simulink model "ADCS_loop"  (R2026a)
settings: Solver=FixedStepDiscrete  StopTime=1500  FixedStep=0.05  EnableMultiTasking=on
undefined symbols (not defined in the file): abs_omega, abs_q, area_of_coil, DiscIntNeverNeededParam, ECI_orbit_positions, k_gain_mag, MOI_tensor, mu_eff, no_of_turns, q_demanded, wheel_omega_initial
libraries: matrix_library x4, dspinverses x1, vrlib x1, dspbuff3 x1
settings Model: Creator=CS  LastModifiedBy=CS
settings SolverCC: AllowMultiTaskInputOutput=on

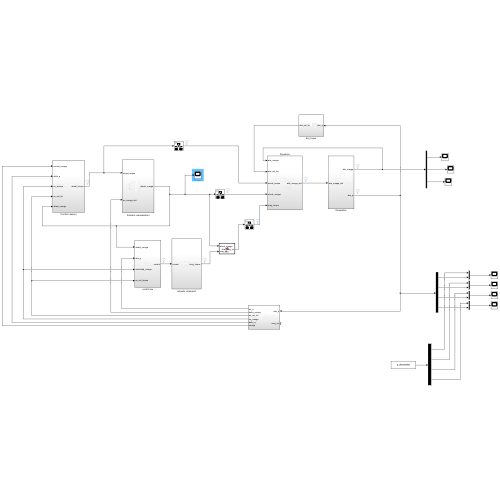
[thumbnail: Simulink's stored preview of the top-level diagram]
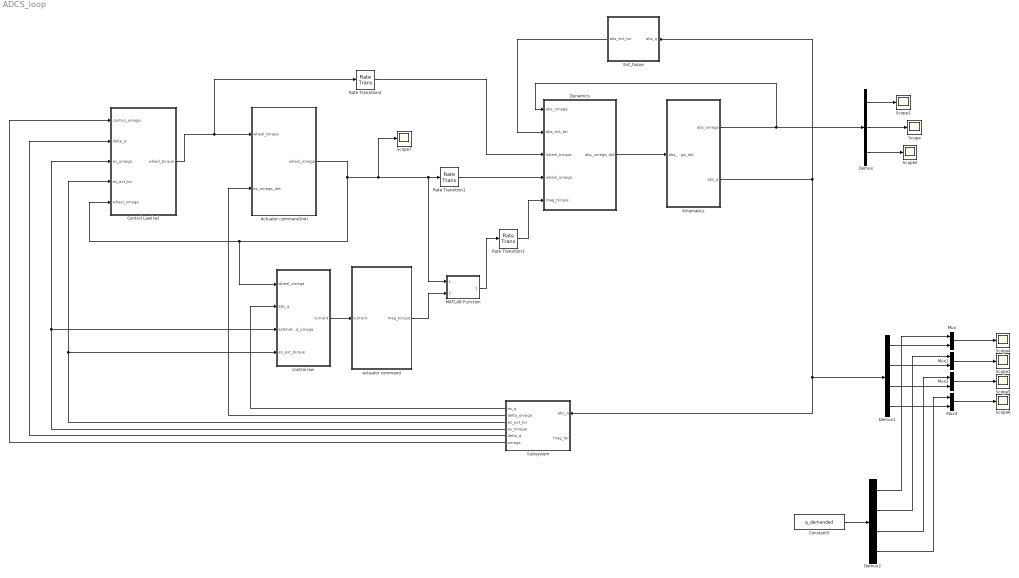
== system ADCS_loop ==
  Actuator command(rw) : Subsystem
  Constant5 : Constant  Value=q_demanded
  Control Law(rw) : Subsystem
  Demux : Demux  Outputs=3
  Demux1 : Demux
  Demux2 : Demux
  Dynamics : Subsystem
  Ext_toque : Subsystem
  Kinematics : Subsystem
  MATLAB Function : MATLAB Function  TreatAsAtomicUnit=on  SystemSampleTime=0.2
  Mux{,1..3} (4 alike) : Mux  Inputs=2
  Rate Transition1 : RateTransition  OutPortSampleTime=0.05
  Rate Transition2 : RateTransition  OutPortSampleTime=0.05
  Rate Transition3 : RateTransition  OutPortSampleTime=0.05
  Scope{,1..7} (8 alike) : Scope
      Scope settings: ActiveDisplayYMinimum=-0.10145714218919644  ActiveDisplayYMaximum=0.1169019272618283
      Scope1 settings: ActiveDisplayYMinimum=-0.0061261723528138138  ActiveDisplayYMaximum=0.0036565085131540572
      Scope2 settings: ActiveDisplayYMinimum=-0.24985187557912408  ActiveDisplayYMaximum=0.81416779259021288  DataLoggingVariableName=ScopeData2
      Scope3 settings: ActiveDisplayYMinimum=-0.0068417213457600129  ActiveDisplayYMaximum=0.0019405957953945842  DataLoggingVariableName=ScopeData3
      Scope4 settings: ActiveDisplayYMinimum=-0.11784086534209379  ActiveDisplayYMaximum=0.16507427528637539  DataLoggingVariableName=ScopeData4
      Scope5 settings: ActiveDisplayYMinimum=0.6667269446379438  ActiveDisplayYMaximum=0.9454278732496123  DataLoggingVariableName=ScopeData5
      Scope6 settings: ActiveDisplayYMinimum=0.44158444098494709  ActiveDisplayYMaximum=0.4580946893794699  DataLoggingVariableName=ScopeData6
      Scope7 settings: ActiveDisplayYMinimum=-2840.1232496648549  ActiveDisplayYMaximum=7000.2332954035792  DataLoggingVariableName=ScopeData7
  Subsystem : Subsystem
  actuator command : Subsystem
  control law : Subsystem
  wires:
  Rate Transition1/1 -> Dynamics/4(wheel_omega)
  Kinematics/2(abs_q) -> Subsystem/1(abs_q), Demux1/1, Ext_toque/1(abs_q)
  Dynamics/1(abs_omega_dot) -> Kinematics/1(abs_omega_dot)
  Kinematics/1(abs_omega) -> Demux/1, Dynamics/1(abs_omega)
  Demux/2 -> Scope/1
  Demux/3 -> Scope2/1
  Demux/1 -> Scope3/1
  Control Law(rw)/1(wheel_torque) -> Rate Transition2/1, Actuator command(rw)/1(wheel_torque)
  Actuator command(rw)/1(wheel_omega) -> control law/1(wheel_omega), Control Law(rw)/5(wheel_omega), Scope7/1, Rate Transition1/1, MATLAB Function/1(wheel_omega)
  Rate Transition2/1 -> Dynamics/3(wheel_torque)
  Constant5/1 -> Demux2/1
  Demux1/1 -> Mux/2
  Demux2/1 -> Mux/1
  Demux1/2 -> Mux1/2
  Demux2/2 -> Mux1/1
  Demux1/3 -> Mux2/2
  Demux2/3 -> Mux2/1
  Mux3/1 -> Scope6/1
  Demux1/4 -> Mux3/2
  Demux2/4 -> Mux3/1
  Mux2/1 -> Scope5/1
  Mux1/1 -> Scope1/1
  Mux/1 -> Scope4/1
  Ext_toque/1(abs_ext_tor) -> Dynamics/2(abs_ext_tor)
  Subsystem/6(omega) -> Control Law(rw)/1(control_omega)
  Subsystem/5(delta_q) -> Control Law(rw)/2(delta_q)
  Subsystem/4(es_omega) -> control law/3(estimated_omega), Control Law(rw)/3(es_omega)
  Subsystem/3(es_ext_tor) -> control law/4(es_ext_torque), Control Law(rw)/4(es_ext_tor)
  Subsystem/2(delta_omega) -> Actuator command(rw)/2(es_omega_dot)
  control law/1(current) -> actuator command/1(current)
  Subsystem/1(es_q) -> control law/2(abs_q)
  actuator command/1(mag_torque) -> MATLAB Function/2(mag_tor)
  Rate Transition3/1 -> Dynamics/5(mag_torque)
  MATLAB Function/1(final_mag_tor) -> Rate Transition3/1

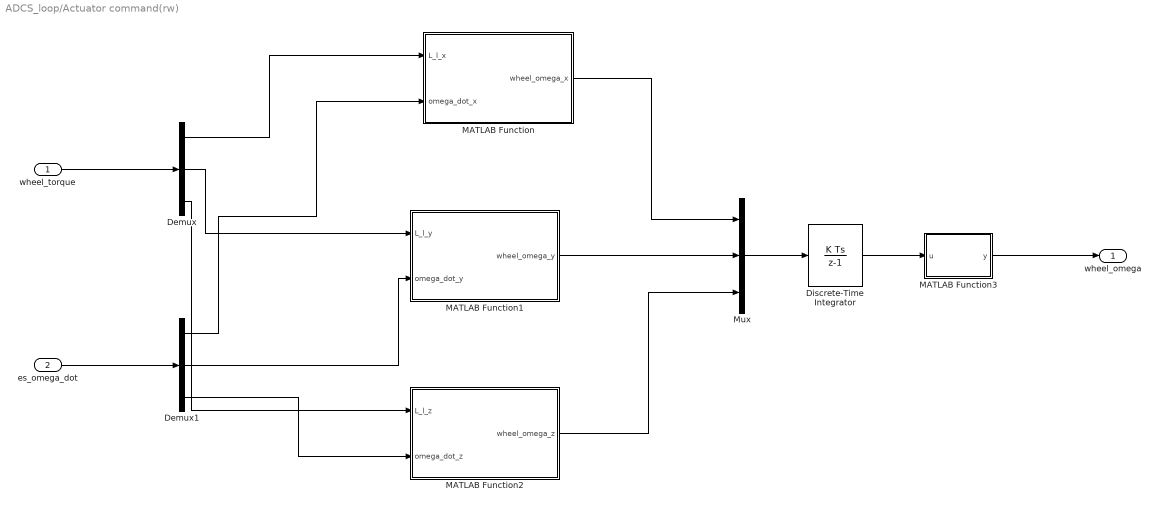
== system ADCS_loop/Actuator command(rw) ==
  wheel_torque : Inport
  es_omega_dot : Inport  Port=2
  Demux : Demux  Outputs=3
  Demux1 : Demux  Outputs=3
  Discrete-Time Integrator : DiscreteIntegrator  InitialCondition=wheel_omega_initial  SampleTime=0.2  ICPrevOutput=DiscIntNeverNeededParam  ICPrevScaledInput=DiscIntNeverNeededParam
  MATLAB Function : MATLAB Function  TreatAsAtomicUnit=on
  MATLAB Function1 : MATLAB Function  TreatAsAtomicUnit=on
  MATLAB Function2 : MATLAB Function  TreatAsAtomicUnit=on
  MATLAB Function3 : MATLAB Function  TreatAsAtomicUnit=on
  Mux : Mux  Inputs=3
  wheel_omega : Outport
  wires:
  wheel_torque/1 -> Demux/1
  es_omega_dot/1 -> Demux1/1
  Demux/1 -> MATLAB Function/1(L_l_x)
  Demux/2 -> MATLAB Function1/1(L_l_y)
  Demux/3 -> MATLAB Function2/1(L_l_z)
  Demux1/1 -> MATLAB Function/2(omega_dot_x)
  Demux1/2 -> MATLAB Function1/2(omega_dot_y)
  Demux1/3 -> MATLAB Function2/2(omega_dot_z)
  MATLAB Function/1(wheel_omega_x) -> Mux/1
  MATLAB Function1/1(wheel_omega_y) -> Mux/2
  MATLAB Function2/1(wheel_omega_z) -> Mux/3
  MATLAB Function3/1(y) -> wheel_omega/1
  Discrete-Time Integrator/1 -> MATLAB Function3/1(u)
  Mux/1 -> Discrete-Time Integrator/1

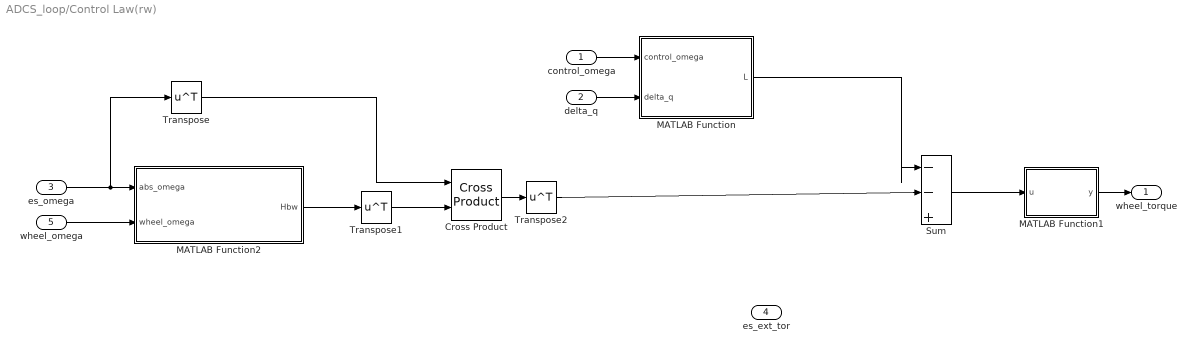
== system ADCS_loop/Control Law(rw) ==
  control_omega : Inport
  delta_q : Inport  Port=2
  es_omega : Inport  Port=3
  es_ext_tor : Inport  Port=4
  wheel_omega : Inport  Port=5
  Cross Product : matrix_library/Cross Product
  MATLAB Function : MATLAB Function  TreatAsAtomicUnit=on  SystemSampleTime=0.2
  MATLAB Function1 : MATLAB Function  TreatAsAtomicUnit=on
  MATLAB Function2 : MATLAB Function  TreatAsAtomicUnit=on  SystemSampleTime=0.2
  Sum : Sum  Inputs=|--+
  Transpose : Math  Operator=transpose
  Transpose1 : Math  Operator=transpose
  Transpose2 : Math  Operator=transpose
  wheel_torque : Outport
  wires:
  delta_q/1 -> MATLAB Function/2(delta_q)
  control_omega/1 -> MATLAB Function/1(control_omega)
  MATLAB Function/1(L) -> Sum/1
  MATLAB Function1/1(y) -> wheel_torque/1
  Sum/1 -> MATLAB Function1/1(u)
  wheel_omega/1 -> MATLAB Function2/2(wheel_omega)
  es_omega/1 -> MATLAB Function2/1(abs_omega), Transpose/1
  MATLAB Function2/1(Hbw) -> Transpose1/1
  Transpose1/1 -> Cross Product/2
  Transpose/1 -> Cross Product/1
  Cross Product/1 -> Transpose2/1
  Transpose2/1 -> Sum/2

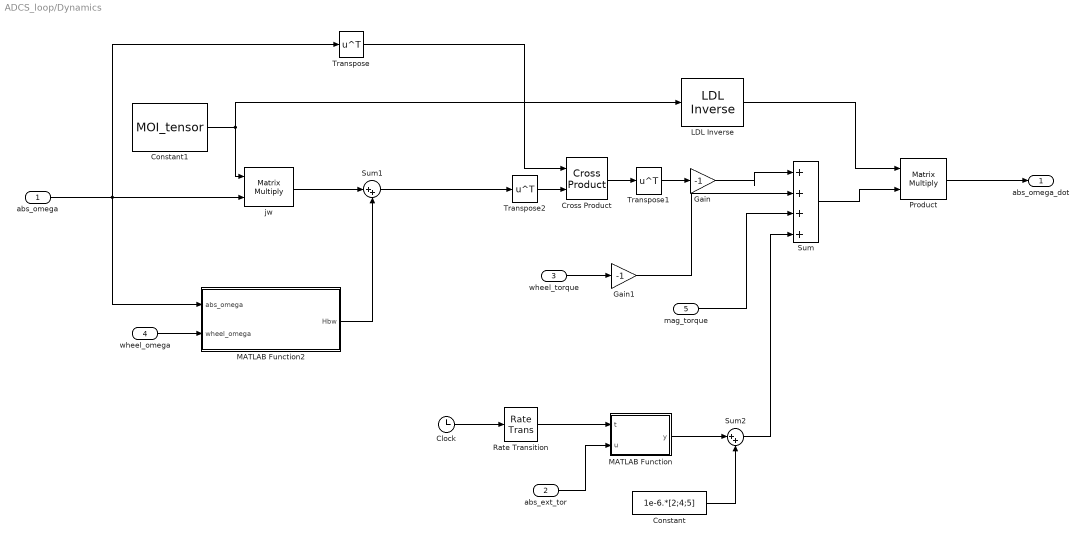
== system ADCS_loop/Dynamics ==
  abs_omega : Inport
  abs_ext_tor : Inport  Port=2
  wheel_torque : Inport  Port=3
  wheel_omega : Inport  Port=4
  mag_torque : Inport  Port=5
  Clock : Clock
  Constant : Constant  Value=1e-6.*[2;4;5]
  Constant1 : Constant  Value=MOI_tensor
  Cross Product : matrix_library/Cross Product
  Gain : Gain  Gain=-1
  Gain1 : Gain  Gain=-1
  LDL Inverse : dspinverses/LDL Inverse  errmode=Warning
  MATLAB Function : MATLAB Function  TreatAsAtomicUnit=on
  MATLAB Function2 : MATLAB Function  TreatAsAtomicUnit=on  SystemSampleTime=0.05
  Product : Product  Multiplication=Matrix(*)
  Rate Transition : RateTransition  OutPortSampleTime=0.05
  Sum : Sum  Inputs=|++++
  Sum1 : Sum  Inputs=|++
  Sum2 : Sum  Inputs=|++
  Transpose : Math  Operator=transpose
  Transpose1 : Math  Operator=transpose
  Transpose2 : Math  Operator=transpose
  jw : Product  Multiplication=Matrix(*)
  abs_omega_dot : Outport
  wires:
  Sum/1 -> Product/2
  LDL Inverse/1 -> Product/1
  Product/1 -> abs_omega_dot/1
  Gain/1 -> Sum/1
  abs_omega/1 -> jw/2, Transpose/1, MATLAB Function2/1(abs_omega)
  Constant1/1 -> LDL Inverse/1, jw/1
  Transpose/1 -> Cross Product/1
  Cross Product/1 -> Transpose1/1
  Transpose1/1 -> Gain/1
  Transpose2/1 -> Cross Product/2
  abs_ext_tor/1 -> MATLAB Function/2(u)
  Rate Transition/1 -> MATLAB Function/1(t)
  Clock/1 -> Rate Transition/1
  wheel_omega/1 -> MATLAB Function2/2(wheel_omega)
  jw/1 -> Sum1/1
  Sum1/1 -> Transpose2/1
  MATLAB Function2/1(Hbw) -> Sum1/2
  mag_torque/1 -> Sum/3
  wheel_torque/1 -> Gain1/1
  Gain1/1 -> Sum/2
  MATLAB Function/1(y) -> Sum2/1
  Sum2/1 -> Sum/4
  Constant/1 -> Sum2/2

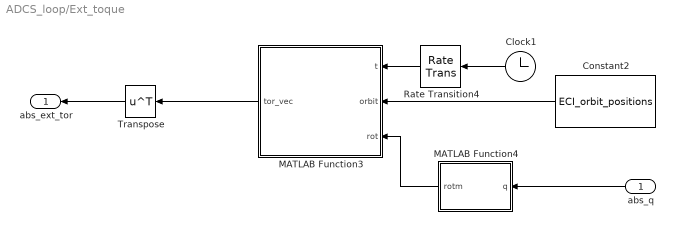
== system ADCS_loop/Ext_toque ==
  abs_q : Inport
  Clock1 : Clock
  Constant2 : Constant  Value=ECI_orbit_positions
  MATLAB Function3 : MATLAB Function  TreatAsAtomicUnit=on
  MATLAB Function4 : MATLAB Function  TreatAsAtomicUnit=on  SystemSampleTime=0.05
  Rate Transition4 : RateTransition  OutPortSampleTime=0.05
  Transpose : Math  Operator=transpose
  abs_ext_tor : Outport
  wires:
  MATLAB Function4/1(rotm) -> MATLAB Function3/3(rot)
  Clock1/1 -> Rate Transition4/1
  MATLAB Function3/1(tor_vec) -> Transpose/1
  Transpose/1 -> abs_ext_tor/1
  abs_q/1 -> MATLAB Function4/1(q)
  Constant2/1 -> MATLAB Function3/2(orbit)
  Rate Transition4/1 -> MATLAB Function3/1(t)

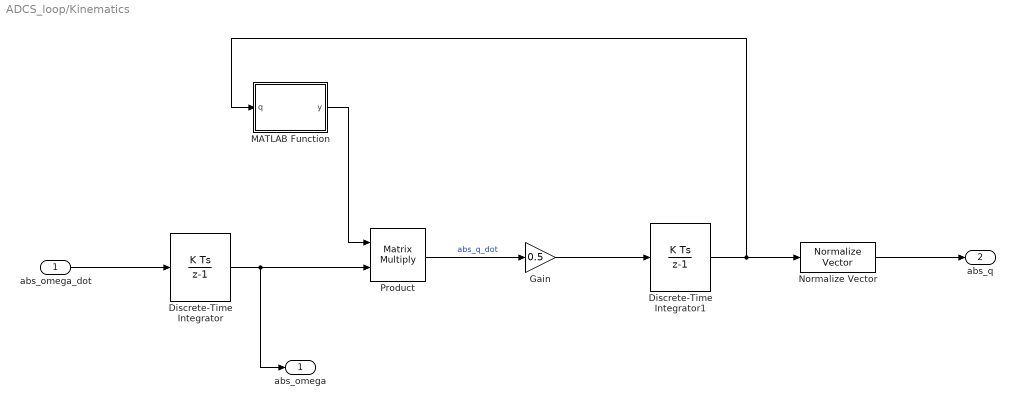
== system ADCS_loop/Kinematics ==
  abs_omega_dot : Inport
  Discrete-Time Integrator : DiscreteIntegrator  InitialCondition=abs_omega  SampleTime=0.05  ICPrevOutput=DiscIntNeverNeededParam  ICPrevScaledInput=DiscIntNeverNeededParam
  Discrete-Time Integrator1 : DiscreteIntegrator  InitialCondition=abs_q  SampleTime=-1  ICPrevOutput=DiscIntNeverNeededParam  ICPrevScaledInput=DiscIntNeverNeededParam
  Gain : Gain  Gain=0.5
  MATLAB Function : MATLAB Function  TreatAsAtomicUnit=on
  Normalize Vector : vrlib/Utilities/Normalize Vector  maxzero=0
  Product : Product  Multiplication=Matrix(*)
  abs_omega : Outport
  abs_q : Outport  Port=2
  wires:
  MATLAB Function/1(y) -> Product/1
  abs_omega_dot/1 -> Discrete-Time Integrator/1
  Discrete-Time Integrator/1 -> Product/2, abs_omega/1
  Product/1 -> Gain/1  "abs_q_dot"
  Discrete-Time Integrator1/1 -> Normalize Vector/1, MATLAB Function/1(q)
  Gain/1 -> Discrete-Time Integrator1/1
  Normalize Vector/1 -> abs_q/1

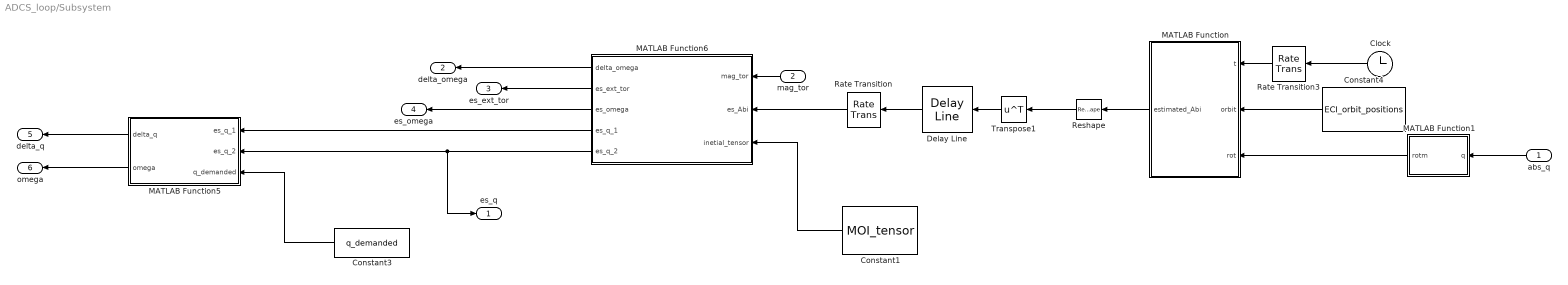
== system ADCS_loop/Subsystem ==
  abs_q : Inport
  mag_tor : Inport  Port=2
  Clock : Clock
  Constant1 : Constant  Value=MOI_tensor
  Constant3 : Constant  Value=q_demanded
  Constant4 : Constant  Value=ECI_orbit_positions
  Delay Line : dspbuff3/Delay Line  siz=4  ic=0  directfeed=off  enable_output=off  hold_output=off  OutputFrames=off
  MATLAB Function : MATLAB Function  TreatAsAtomicUnit=on  SystemSampleTime=0.05
  MATLAB Function1 : MATLAB Function  TreatAsAtomicUnit=on  SystemSampleTime=0.05
  MATLAB Function5 : MATLAB Function  TreatAsAtomicUnit=on  SystemSampleTime=0.2
  MATLAB Function6 : MATLAB Function  TreatAsAtomicUnit=on  SystemSampleTime=0.2
  Rate Transition : RateTransition  OutPortSampleTime=0.2
  Rate Transition3 : RateTransition  OutPortSampleTime=0.05
  Reshape : Reshape  OutputDimensionality=Customize  OutputDimensions=[9,1]
  Transpose1 : Math  Operator=transpose
  es_q : Outport
  delta_omega : Outport  Port=2
  es_ext_tor : Outport  Port=3
  es_omega : Outport  Port=4
  delta_q : Outport  Port=5
  omega : Outport  Port=6
  wires:
  Transpose1/1 -> Delay Line/1
  MATLAB Function6/2(es_ext_tor) -> es_ext_tor/1
  MATLAB Function/1(estimated_Abi) -> Reshape/1
  Constant4/1 -> MATLAB Function/2(orbit)
  mag_tor/1 -> MATLAB Function6/1(mag_tor)
  MATLAB Function1/1(rotm) -> MATLAB Function/3(rot)
  Clock/1 -> Rate Transition3/1
  MATLAB Function6/5(es_q_2) -> es_q/1, MATLAB Function5/2(es_q_2)
  Rate Transition3/1 -> MATLAB Function/1(t)
  MATLAB Function6/3(es_omega) -> es_omega/1
  MATLAB Function6/4(es_q_1) -> MATLAB Function5/1(es_q_1)
  Constant3/1 -> MATLAB Function5/3(q_demanded)
  Constant1/1 -> MATLAB Function6/3(inetial_tensor)
  Rate Transition/1 -> MATLAB Function6/2(es_Abi)
  Reshape/1 -> Transpose1/1
  Delay Line/1 -> Rate Transition/1
  MATLAB Function6/1(delta_omega) -> delta_omega/1
  abs_q/1 -> MATLAB Function1/1(q)
  MATLAB Function5/1(delta_q) -> delta_q/1
  MATLAB Function5/2(omega) -> omega/1

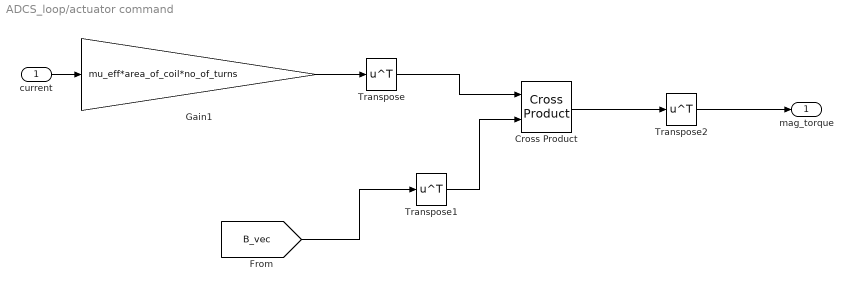
== system ADCS_loop/actuator command ==
  current : Inport
  Cross Product : matrix_library/Cross Product
  Gain1 : Gain  Gain=mu_eff*area_of_coil*no_of_turns
  Transpose : Math  Operator=transpose
  Transpose1 : Math  Operator=transpose
  Transpose2 : Math  Operator=transpose
  mag_torque : Outport
  wires:
  current/1 -> Gain1/1
  Gain1/1 -> Transpose/1
  [B_vec] -> Transpose1/1
  Transpose1/1 -> Cross Product/2
  Transpose/1 -> Cross Product/1
  Cross Product/1 -> Transpose2/1
  Transpose2/1 -> mag_torque/1

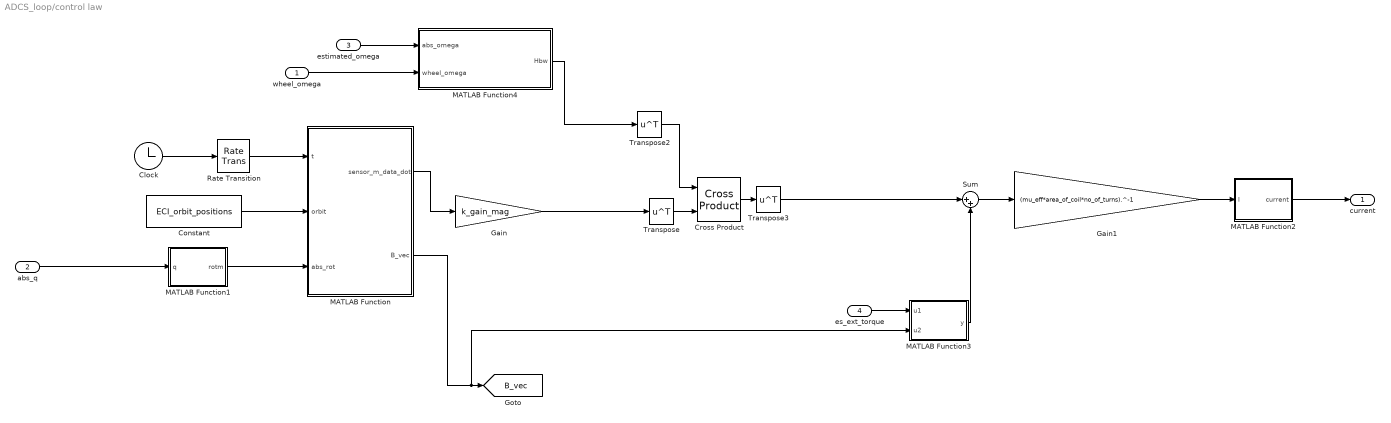
== system ADCS_loop/control law ==
  wheel_omega : Inport
  abs_q : Inport  Port=2
  estimated_omega : Inport  Port=3
  es_ext_torque : Inport  Port=4
  Clock : Clock
      settings: Decimation=200
  Constant : Constant  Value=ECI_orbit_positions
  Cross Product : matrix_library/Cross Product
  Gain : Gain  Gain=k_gain_mag
  Gain1 : Gain  Gain=(mu_eff*area_of_coil*no_of_turns).^-1
  MATLAB Function : MATLAB Function  TreatAsAtomicUnit=on  SystemSampleTime=0.2
  MATLAB Function1 : MATLAB Function  TreatAsAtomicUnit=on  SystemSampleTime=0.2
  MATLAB Function2 : MATLAB Function  TreatAsAtomicUnit=on  SystemSampleTime=0.2
  MATLAB Function3 : MATLAB Function  TreatAsAtomicUnit=on
  MATLAB Function4 : MATLAB Function  TreatAsAtomicUnit=on  SystemSampleTime=0.2
  Rate Transition : RateTransition  OutPortSampleTime=0.2
  Sum : Sum  Inputs=|++
  Transpose : Math  Operator=transpose
  Transpose2 : Math  Operator=transpose
  Transpose3 : Math  Operator=transpose
  current : Outport
  tag scope: B_vec=global
  wires:
  Constant/1 -> MATLAB Function/2(orbit)
  MATLAB Function1/1(rotm) -> MATLAB Function/3(abs_rot)
  MATLAB Function/1(sensor_m_data_dot) -> Gain/1
  abs_q/1 -> MATLAB Function1/1(q)
  Transpose2/1 -> Cross Product/1
  Cross Product/1 -> Transpose3/1
  Gain1/1 -> MATLAB Function2/1(I)
  MATLAB Function2/1(current) -> current/1
  MATLAB Function/2(B_vec) -> MATLAB Function3/2(u2), [B_vec]
  Sum/1 -> Gain1/1
  Rate Transition/1 -> MATLAB Function/1(t)
  Clock/1 -> Rate Transition/1
  Transpose/1 -> Cross Product/2
  Gain/1 -> Transpose/1
  es_ext_torque/1 -> MATLAB Function3/1(u1)
  MATLAB Function3/1(y) -> Sum/2
  Transpose3/1 -> Sum/1
  estimated_omega/1 -> MATLAB Function4/1(abs_omega)
  wheel_omega/1 -> MATLAB Function4/2(wheel_omega)
  MATLAB Function4/1(Hbw) -> Transpose2/1

== matlab function ADCS_loop/Actuator command(rw)/MATLAB Function2 ==
  data: L_l_z input; wheel_omega_z output; omega_dot_z input
function wheel_omega_z = wheel_omega_final_z(L_l_z,omega_dot_z)

wheel_omega_z = ((L_l_z/(1e-7*9.37)) - omega_dot_z);

== matlab function ADCS_loop/Actuator command(rw)/MATLAB Function3 ==
  data: u input; y output
function y = fcn(u)
y=[0;0;0];
if -5696 < u(1) && u(1)<5969
    y(1) = u(1);
elseif u(1)<-5696
    y(1) = -5696;
else
    y(1) = 5969;
end
if -5696 < u(2) && u(2)<5969
    y(2) = u(2);
elseif u(2)<-5696
    y(2) = -5696;
else
    y(2) = 5969;
end
if -5696 < u(3) && u(3)<5969
    y(3) = u(3);
elseif u(3)<-5696
    y(3) = -5696;
else
    y(3) = 5969;
end

== matlab function ADCS_loop/Subsystem/MATLAB Function5 ==
  data: es_q_1 input; es_q_2 input; q_demanded input; delta_q output; omega output
function [delta_q,omega] = delta(es_q_1,es_q_2,q_demanded)
q1 =q_demanded(1);
q2 =q_demanded(2);
q3 =q_demanded(3);
q4 =q_demanded(4);
y =[q4,-q3,q2;q3,q4,-q1;-q2,q1,q4;-q1,-q2,-q3];
delta_q_vec_1 = y'*es_q_1;
delta_q_4_1 = es_q_1'*q_demanded;
delta_q_1 = [delta_q_vec_1(1);delta_q_vec_1(2);delta_q_vec_1(3);delta_q_4_1];
delta_q_vec_2 = y'*es_q_2;
delta_q_4_2 = es_q_2'*q_demanded;
delta_q = [delta_q_vec_2(1);delta_q_vec_2(2);delta_q_vec_2(3);delta_q_4_2];
delta_q_dot = 20.*(delta_q - delta_q_1);
A = [delta_q_1(4),-1*delta_q_1(3),delta_q_1(2);delta_q_1(3),delta_q_1(4),-1*delta_q_1(1);-1*delta_q_1(2),delta_q_1(1),delta_q_1(4)];
B = [delta_q_dot(1);delta_q_dot(2);delta_q_dot(3)];
omega = A\B;

== matlab function ADCS_loop/Control Law(rw)/MATLAB Function ==
  data: control_omega input; L output; delta_q input
   function L = control_torque(control_omega,delta_q)
Kp =0.0075;
Kd = 0.0175;
L = (-1*Kp*sign(delta_q(4))).*[delta_q(1);delta_q(2);delta_q(3)] - Kd.*control_omega;

== matlab function ADCS_loop/Control Law(rw)/MATLAB Function2 ==
  data: abs_omega input; Hbw output; wheel_omega input
function Hbw = H_b_w(abs_omega,wheel_omega)

Hbw_x = 1e-7*9.37*(abs_omega(1)+wheel_omega(1));
Hbw_y = 1e-7*9.37*(abs_omega(2)+wheel_omega(2));
Hbw_z = 1e-7*9.37*(abs_omega(3)+wheel_omega(3));
Hbw = [Hbw_x;Hbw_y;Hbw_z];

== matlab function ADCS_loop/Dynamics/MATLAB Function2 ==
  data: abs_omega input; Hbw output; wheel_omega input
function Hbw = H_b_w(abs_omega,wheel_omega)
Hbw_x = 1e-7*9.37*(abs_omega(1)+wheel_omega(1));
Hbw_y = 1e-7*9.37*(abs_omega(2)+wheel_omega(2));
Hbw_z = 1e-7*9.37*(abs_omega(3)+wheel_omega(3));
Hbw = [Hbw_x;Hbw_y;Hbw_z];

== matlab function ADCS_loop/control law/MATLAB Function ==
  settings: updateMethod=DISCRETE
  data: t input; sensor_m_data_dot output; orbit input; abs_rot input; B_vec output
function [sensor_m_data_dot,B_vec]= b_vector(t,orbit,abs_rot)
tu2 = t/0.05;
tu = round(tu2);
T = tu+ 40000;
current_pos_xyz = orbit(T,:);
current_pos_xyz = current_pos_xyz/norm(current_pos_xyz);
theta = asind(current_pos_xyz(3));
LST = atan2d(current_pos_xyz(2), current_pos_xyz(1));% range:[0,pi/2]
Re = 6.37814e+3; 
Y = 2026;
M = 3;
D = 20;
s=t;
m=0;
h=0;
m = floor(s / 60);
s = mod(s, 60);
h = floor(m / 60);
m = mod(m, 60);
JD = 367*Y - floor((7/4)*(Y+floor((M+9)/12))) + floor(275*M/9) + D + 1721013.5;
Tut1 = (JD-2541545.0)/36525;
theta_gmst = 24110.54841+ 8640184.812866*Tut1+ 0.093104*(Tut1).^2 - 6.2*(10.^-6)*(Tut1.^3) + 1.002737909350795*(3600*h + 60*m+s);
theta_gmst = theta_gmst - 86400*(floor(theta_gmst/86400));
theta_gmst = theta_gmst/240;
phi = 360 + (LST-theta_gmst);
phi = mod(phi, 360); % Normalize phi to the range [0, 360]
sensor_m_data1 = magnetometer_sensor(Re,theta,phi,9574,Y,M,D,h,m,s,abs_rot);
% sensor_m_data2 = magnetometer_sensor(Re,theta,phi,9574,Y,M,D,h,m,s+1,abs_rot);
B_vec = sensor_m_data1';
sensor_m_data_dot = sensor_m_data1/norm(sensor_m_data1);
sensor_m_data_dot = sensor_m_data_dot'./norm(sensor_m_data1);

== matlab function ADCS_loop/control law/MATLAB Function1 ==
  data: q input; rotm output
function rotm  = Quat_to_rotm(q)
% Normalize the quaternion
q = q / norm(q);
% Extract the components of the quaternion
q1 = q(1,1);
q2 = q(2,1);
q3 = q(3,1);
q4 = q(4,1);

% Compute the rotation matrix
rotm = [1 - 2*(q2^2 + q3^2), 2*(q1*q2 + q3*q4), 2*(q1*q3 - q2*q4);
    2*(q1*q2 - q3*q4), 1 - 2*(q1^2 + q3^2), 2*(q2*q3 + q1*q4);
    2*(q1*q3 + q2*q4), 2*(q2*q3 - q1*q4), 1 - 2*(q1^2 + q2^2)];

== matlab function ADCS_loop/control law/MATLAB Function2 ==
  data: I input; current output
function current = limit_check(I)
current = [0;0;0];
if I(1,1)<0.1 && I(1,1)>-0.1
    current(1,1)=I(1,1);
elseif I(1,1)>0.1
    current(1,1)=0.1;
else
    current(1,1)=-0.1;
end
if I(2,1)<0.1 && I(2,1)>-0.1
    current(2,1)=I(2,1);
elseif I(2,1)>0.1
    current(2,1)=0.1;
else
    current(2,1)=-0.1;
end

if I(3,1)<0.1 && I(3,1)>-0.1
    current(3,1)=I(3,1);
elseif I(3,1)>0.1
    current(3,1)=0.1;
else
    current(3,1)=-0.1;
end

== matlab function ADCS_loop/control law/MATLAB Function3 ==
  data: u1 input; y output; u2 input
function y = fcn(u1,u2)


y = u1/norm(u2);

== matlab function ADCS_loop/Kinematics/MATLAB Function ==
  data: q input; y output
function y = quat_dot_matrix(q)
q1 =q(1);
q2 =q(2);
q3 =q(3);
q4 =q(4);
y =[q4,-q3,q2;q3,q4,-q1;-q2,q1,q4;-q1,-q2,-q3];

== matlab function ADCS_loop/control law/MATLAB Function4 ==
  data: abs_omega input; Hbw output; wheel_omega input
function Hbw = H_b_w(abs_omega,wheel_omega)

Hbw_x = 1e-7*9.37*(abs_omega(1)+wheel_omega(1));
Hbw_y = 1e-7*9.37*(abs_omega(2)+wheel_omega(2));
Hbw_z = 1e-7*9.37*(abs_omega(3)+wheel_omega(3));
Hbw = [Hbw_x;Hbw_y;Hbw_z];

== matlab function ADCS_loop/MATLAB Function ==
  data: wheel_omega input; final_mag_tor output; mag_tor input
function final_mag_tor = fcn(wheel_omega,mag_tor)
persistent status;
final_mag_tor = [0;0;0];
if isempty(status)
    status = 0;
end
if wheel_omega(1) > 5000 || wheel_omega(1) < -5000 || wheel_omega(2) > 5000 || wheel_omega(2) < -5000 || wheel_omega(3) > 5000 || wheel_omega(3) < -5000
    status = 1;
end
if -500<wheel_omega(1) && wheel_omega(1) < 500 || -500<wheel_omega(2) && wheel_omega(2) < 500 || -500<wheel_omega(3) && wheel_omega(3) < 500
    status = 0;
end
if status == 1
    final_mag_tor = mag_tor;
end
if status == 0
    final_mag_tor = [0;0;0];
end

== matlab function ADCS_loop/Subsystem/MATLAB Function6 ==
  data: delta_omega output; mag_tor input; es_Abi input; es_ext_tor output; es_omega output; es_q_1 output; inetial_tensor input; es_q_2 output
function [delta_omega,es_ext_tor,es_omega,es_q_1,es_q_2]= acc__omega(mag_tor,es_Abi,inetial_tensor)
es1=[es_Abi(1,1) es_Abi(1,4) es_Abi(1,7);es_Abi(1,2) es_Abi(1,5) es_Abi(1,8);es_Abi(1,3) es_Abi(1,6) es_Abi(1,9)];
es2=[es_Abi(2,1) es_Abi(2,4) es_Abi(2,7);es_Abi(2,2) es_Abi(2,5) es_Abi(2,8);es_Abi(2,3) es_Abi(2,6) es_Abi(2,9)];
es3=[es_Abi(3,1) es_Abi(3,4) es_Abi(3,7);es_Abi(3,2) es_Abi(3,5) es_Abi(3,8);es_Abi(3,3) es_Abi(3,6) es_Abi(3,9)];
es4=[es_Abi(4,1) es_Abi(4,4) es_Abi(4,7);es_Abi(4,2) es_Abi(4,5) es_Abi(4,8);es_Abi(4,3) es_Abi(4,6) es_Abi(4,9)];
q1 = rotm2quat(es1);
temp = q1;
q1 = [-temp(2);-temp(3);-temp(4);temp(1)];
q2 = rotm2quat(es2);
temp = q2;
q2 = [-temp(2);-temp(3);-temp(4);temp(1)];
q3 = rotm2quat(es3);
temp = q3;
q3 = [-temp(2);-temp(3);-temp(4);temp(1)];
q4 = rotm2quat(es4);
temp = q4;
q4 = [-temp(2);-temp(3);-temp(4);temp(1)];
q1_dot = 20.*(q2-q1);
q3_dot = 20.*(q4-q3);
% y =[q4,-q3,q2;q3,q4,-q1;-q2,q1,q4;-q1,-q2,-q3];
y1 = [q1(4),q1(3),-q1(2),-q1(1);-q1(3),q1(4),q1(1),-q1(2);q1(2),-q1(1),q1(4),-q1(3)];
y2 = [q3(4),q3(3),-q3(2),-q3(1);-q3(3),q3(4),q3(1),-q3(2);q3(2),-q3(1),q3(4),-q3(3)];
w1 = 2.*(y1*q1_dot);
w2 = 2.*(y2*q3_dot);
es_omega = w2;
delta_omega = 20.*(w2 - w1);
jw_dot = inetial_tensor*delta_omega;
jw = inetial_tensor*w2;
wxjw = cross(w2' , jw');
wxjw = wxjw';
es_ext_tor = 1e-3.*(jw_dot + wxjw - mag_tor);
es_q_1 = q3;
es_q_2 = q4;

== matlab function ADCS_loop/Control Law(rw)/MATLAB Function1 ==
  data: u input; y output
function y = fcn(u)
y=[0;0;0];
if -0.00097 < u(1) && u(1)<0.00097
    y(1) = u(1);
elseif u(1)<-0.00097
    y(1) = -0.00097;
else
    y(1) =0.00097;
end
if -0.00097 < u(2) && u(2)<0.00097
    y(2) = u(2);
elseif u(2)<-0.00097
    y(2) = -0.00097;
else
    y(2) = 0.00097;
end
if -0.00097< u(3) && u(3)<0.00097
    y(3) = u(3);
elseif u(3)<-0.00097
    y(3) = -0.00097;
else
    y(3) = 0.00097;
end

== matlab function ADCS_loop/Subsystem/MATLAB Function ==
  data: t input; estimated_Abi output; orbit input; rot input
function estimated_Abi  = TRIAD(t,orbit,rot)
tu2 = t/0.05;
tu = round(tu2);
T = tu+ 40000;
current_pos_xyz = orbit(T,:);
current_pos_xyz = current_pos_xyz/norm(current_pos_xyz);
theta = asind(current_pos_xyz(3));
LST = atan2d(current_pos_xyz(2), current_pos_xyz(1));% range:[0,pi/2]
Re = 6.37814e+3; 
Y = 2026;
M = 3;
D = 20;
s=t;
m=0;
h=0;
m = floor(s / 60);
s = mod(s, 60);
h = floor(m / 60);
m = mod(m, 60);
JD = 367*Y - floor((7/4)*(Y+floor((M+9)/12))) + floor(275*M/9) + D + 1721013.5;
Tut1 = (JD-2541545.0)/36525;
theta_gmst = 24110.54841+ 8640184.812866*Tut1+ 0.093104*(Tut1).^2 - 6.2*(10.^-6)*(Tut1.^3) + 1.002737909350795*(3600*h + 60*m+s);
theta_gmst = theta_gmst - 86400*(floor(theta_gmst/86400));
theta_gmst = theta_gmst/240;
phi = 360 + (LST-theta_gmst);
phi = mod(phi, 360); % Normalize phi to the range [0, 360]
m_vector = m_vector_ECI(Re,theta,phi,9574,Y,M,D,h,m,s);
s_vector= Sun_vector_ECI(Y,M,D,h,m,s);
sensor_m_data = magnetometer_sensor(Re,theta,phi,9574,Y,M,D,h,m,s,rot);
s_meas = sensor_m_data;
% Persistent filtered vector
persistent hat

alpha = 0.46;

% New measurement s_meas (3x1)
s_meas = s_meas / norm(s_meas);

if isempty(hat)
    hat = s_meas;
else
    hat = alpha.*s_meas + (1-alpha).*hat;
    hat = hat / norm(hat);
end
sensor_m_data = hat;
sensor_s_data = Sun_sensor(Y,M,D,h,m,s,rot);
s_meas = sensor_s_data;
% Persistent filtered vector
persistent s_hat

alpha = 0.46;

% New measurement s_meas (3x1)
s_meas = s_meas / norm(s_meas);

if isempty(s_hat)
    s_hat = s_meas;
else
    s_hat = alpha.*s_meas + (1-alpha).*s_hat;
    s_hat = s_hat / norm(s_hat);
end
sensor_s_data = s_hat;
t1_B = sensor_s_data;
t2_B = cross(sensor_s_data,sensor_m_data)/norm(cross(sensor_s_data,sensor_m_data));
t3_B = cross(t1_B,t2_B)/norm(cross(t1_B,t2_B));
Abt = [t1_B' t2_B' t3_B'];
t1_N = s_vector;
t2_N = cross(s_vector,m_vector)/norm(cross(s_vector,m_vector));
t3_N = cross(t1_N,t2_N)/norm(cross(t1_N,t2_N));
Ant = [t1_N' t2_N' t3_N'];
estimated_Abi = Abt * Ant'; % Calculate the estimated attitude using the transformation

== matlab function ADCS_loop/Subsystem/MATLAB Function1 ==
  data: q input; rotm output
function rotm  = Quat_to_rotm(q)
% Normalize the quaternion
q = q / norm(q);
% Extract the components of the quaternion
q1 = q(1,1);
q2 = q(2,1);
q3 = q(3,1);
q4 = q(4,1);

% Compute the rotation matrix
rotm = [1 - 2*(q2^2 + q3^2), 2*(q1*q2 + q3*q4), 2*(q1*q3 - q2*q4);
    2*(q1*q2 - q3*q4), 1 - 2*(q1^2 + q3^2), 2*(q2*q3 + q1*q4);
    2*(q1*q3 + q2*q4), 2*(q2*q3 - q1*q4), 1 - 2*(q1^2 + q2^2)];

== matlab function ADCS_loop/Actuator command(rw)/MATLAB Function ==
  data: L_l_x input; wheel_omega_x output; omega_dot_x input
function wheel_omega_x = wheel_omega_final_x(L_l_x,omega_dot_x)
wheel_omega_x = ((L_l_x/(1e-7*9.37)) - omega_dot_x);

== matlab function ADCS_loop/Actuator command(rw)/MATLAB Function1 ==
  data: L_l_y input; wheel_omega_y output; omega_dot_y input
function wheel_omega_y = wheel_omega_final_y(L_l_y,omega_dot_y)

wheel_omega_y = ((L_l_y/(1e-7*9.37)) - omega_dot_y);

== matlab function ADCS_loop/Ext_toque/MATLAB Function3 ==
  data: t input; tor_vec output; orbit input; rot input
function tor_vec  = ext_torque(t,orbit,rot)
Y = 2026;
M = 3;
D = 20;
s=t;
m=0;
h=0;
m = floor(s / 60);
s = mod(s, 60);
h = floor(m / 60);
m = mod(m, 60);
net_torque = zeros(1,3);
surface_area = 3.1584e-6;
N=4;
n1_b = [1 0 0];
n2_b = [0 1 0];
n3_b = [-1 0 0];
n4_b = [0 -1 0];
n_b = [n1_b;n2_b;n3_b;n4_b];
r1_b = [-0.05 0.1 0];
r2_b = [-0.1 -0.05 0];
r3_b = [0.05 -0.1 0];
r4_b = [0.1 0.05 0];
r_b  = [r1_b;r2_b;r3_b;r4_b];
s_ECI = Sun_vector_ECI(Y,M,D,h,m,s);
s_vec = rot*s_ECI';
s_vec = s_vec';
w = 0.000072921158553;
tu2 = t/0.05;
tu = round(tu2);
T = tu+ 40000;
dR = 20.*(orbit(T+1,:) - orbit(T,:));
dr = rot*dR';
dr= dr';
vrel_b=[dr(1)+(w*orbit(T,2)),dr(2)-(w*orbit(T,1)),dr(3)];
for i = 1:N
    cos_aero= dot(n_b(i,:),vrel_b)/norm(vrel_b);
    cos_srp = dot(n_b(i,:),s_vec);
    u = max(cos_aero,0);
    u2 = max(cos_srp,0);
    F_aero = (-0.5*u*norm(vrel_b)*6e-13*1000*2.2).*vrel_b;
    F_srp = (-4.54e-6*surface_area*u2*1000).*((2*(0.04+0.18*cos_srp).*n_b(i,:))+(0.82.*s_vec));
    L_aero = cross(r_b(i,:),F_aero);
    L_srp = cross(r_b(i,:),F_srp);
    net_torque = net_torque + L_aero+L_srp;
end
rand_tor = zeros(1, 3); % Initialize the estimated_Abi matrix
for r = 1:3
        a = -0.02;
        b = 0.03;
        n = 1;
        t = a + (b-a).*rand(n,1);
        rand_tor(1,r) = t*1e-6;
end

tor_vec = net_torque +rand_tor;

== matlab function ADCS_loop/Ext_toque/MATLAB Function4 ==
  data: q input; rotm output
function rotm  = Quat_to_rotm(q)
% Normalize the quaternion
q = q / norm(q);
% Extract the components of the quaternion
q1 = q(1,1);
q2 = q(2,1);
q3 = q(3,1);
q4 = q(4,1);

% Compute the rotation matrix
rotm = [1 - 2*(q2^2 + q3^2), 2*(q1*q2 + q3*q4), 2*(q1*q3 - q2*q4);
    2*(q1*q2 - q3*q4), 1 - 2*(q1^2 + q3^2), 2*(q2*q3 + q1*q4);
    2*(q1*q3 + q2*q4), 2*(q2*q3 - q1*q4), 1 - 2*(q1^2 + q2^2)];

== matlab function ADCS_loop/Dynamics/MATLAB Function ==
  data: t input; u input; y output
function y = fcn(t,u)
if 200<t && t<210
    y=u;
else
    y= [0;0;0];
end
end
